simulink model "basicbpskreceiver"  (R2021a)
settings: Solver=VariableStepAuto  StartTime=0.0  StopTime=1000.0  RelTol=1e-3
libraries: dsp_blocks x7
settings Model: Creator=nathanalemayehu  LastModifiedBy=nathanalemayehu

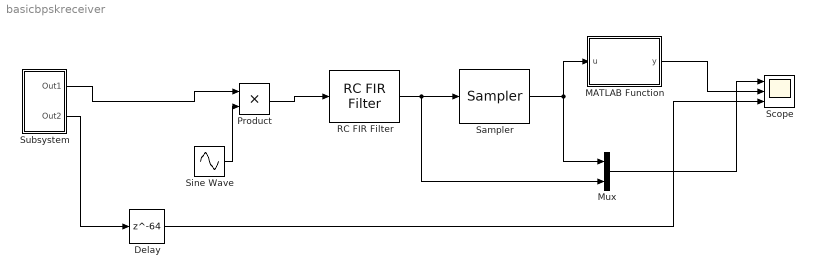
== system basicbpskreceiver ==
  Delay : Delay  DelayLength=64
  MATLAB Function : MATLAB Function  TreatAsAtomicUnit=on
  Mux : Mux  Inputs=2
  Product : Product
  RC FIR Filter : dsp_blocks/Filters/RC FIR Filter  period=50  beta=0.5  root=off  filt_len=128  win_type=off
  Sampler : dsp_blocks/Conversions/Sampler  offset=80  samp_period=50
  Scope : Scope  NumInputPorts=3
  Sine Wave : Sin  Amplitude=2  SampleTime=0
  Subsystem : Subsystem
  wires:
  Subsystem/1(Out1) -> Product/1
  Subsystem/2(Out2) -> Delay/1
  Sine Wave/1 -> Product/2
  Product/1 -> RC FIR Filter/1
  RC FIR Filter/1 -> Mux/2, Sampler/1
  Sampler/1 -> MATLAB Function/1(u), Mux/1
  Mux/1 -> Scope/1
  MATLAB Function/1(y) -> Scope/2
  Delay/1 -> Scope/3

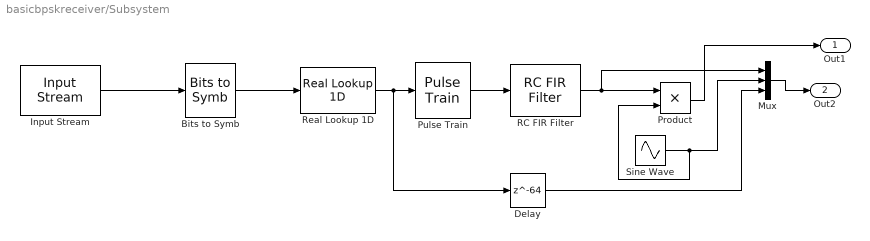
== system basicbpskreceiver/Subsystem ==
  Bits to Symb : dsp_blocks/Conversions/Bits to Symb
  Delay : Delay  DelayLength=64
  Input Stream : dsp_blocks/Sources//Sinks/Input Stream  period=50  width=1  fname=rand.mat
  Mux : Mux  Inputs=3
  Product : Product
  Pulse Train : dsp_blocks/Conversions/Pulse Train  period=50
  RC FIR Filter : dsp_blocks/Filters/RC FIR Filter  period=50  beta=0.5  root=off  filt_len=128  win_type=on
  Real Lookup 1D : dsp_blocks/Conversions/Real Lookup 1D  table=[-1 1]
  Sine Wave : Sin  SampleTime=0
  Out1 : Outport
  Out2 : Outport  Port=2
  wires:
  Input Stream/1 -> Bits to Symb/1
  Bits to Symb/1 -> Real Lookup 1D/1
  Product/1 -> Out1/1
  Sine Wave/1 -> Mux/2, Product/2
  Pulse Train/1 -> RC FIR Filter/1
  Mux/1 -> Out2/1
  Real Lookup 1D/1 -> Delay/1, Pulse Train/1
  Delay/1 -> Mux/3
  RC FIR Filter/1 -> Mux/1, Product/1

== matlab function basicbpskreceiver/MATLAB Function ==
  data: u input; y output
function y = fcn(u)
if(u > 0),
    y = 1;
else 
    y = 0;
end
